simulink model "LR4_MostKran_1"  (R2019b)
settings: Solver=FixedStepAuto  StartTime=0.0  StopTime=70  FixedStep=dT  RelTol=1e-3  EnableMultiTasking=on
values from neighbouring files (symbols this model uses):
  A = [0, 1, 0, 0;  0, 0, a23, 0;  0, 0, 0, 1;  0, 0, a43, 0]    [LR_4_MostKran.m]
  B = [0; b2; 0; b4]    [LR_4_MostKran.m]
  C = [1, 0, 0, 0; 0, 1, 0, 0; 0, 0, 1, 0; 0, 0, 0, 1]    [LR_4_MostKran.m]
  D = [0; 0; 0; 0]    [LR_4_MostKran.m]
  fisREG = readfis('RgMostKran_1')    [LR_4_MostKran.m]
  KdE = 1/3    (= 0.333333333333)    [LR_4_MostKran.m]
  KEr = 1/40    (= 0.025)    [LR_4_MostKran.m]
  KU = 40    [LR_4_MostKran.m]
  X0 = [0; 0; 0; 0]    [LR_4_MostKran.m]
undefined symbols (not defined in the file or in its folder): sigbuilder_block
libraries: fuzblock x1
settings Model: Creator=Сергей  LastModifiedBy=danil
settings DataIOCC: LimitDataPoints=on  ReturnWorkspaceOutputs=off
settings OptimizationCC: LifeSpan=inf
settings DebuggingCC: AllowSymbolicDim=off  SFUnexpectedBacktrackingDiag=warning  SFNoUnconditionalDefaultTransitionDiag=warning  SFExecutionAtInitializationDiag=none  ArithmeticOperatorsInVariantConditions=warning
settings ModelReferenceCC: PropagateSignalLabelsOutOfModel=off
settings SFSimCC: SimUseLocalCustomCode=off  CustomCodeUndefinedFunction=UseInterfaceOnly
settings RTWCC: RTWUseLocalCustomCode=off
settings CodeAppCC: StateflowObjectComments=on
settings GRTTargetCC: TargetLangStandard=C89/C90 (ANSI)
settings ConfigComp: CovMetricSettings=dw  CovHtmlReporting=on  CovSaveCumulativeToWorkspaceVar=on  CovSaveSingleToWorkspaceVar=on  CovExternalEMLEnable=off

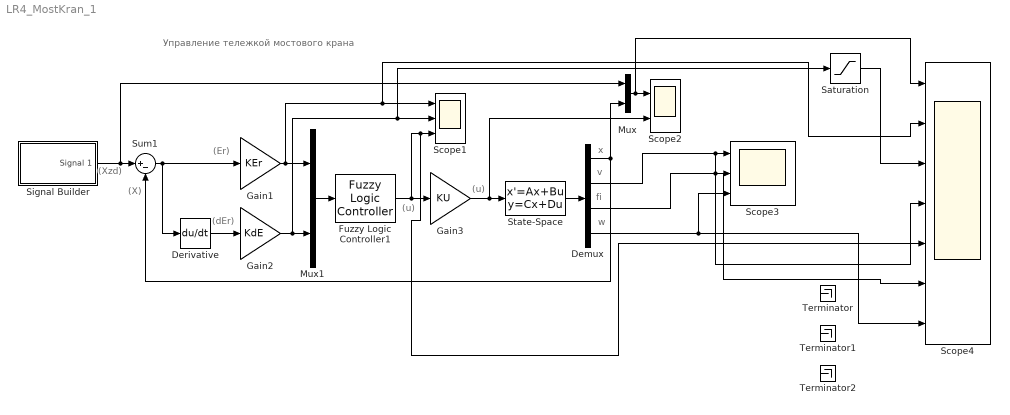
== system LR4_MostKran_1 ==
  note: w
  note: fi
  note: v
  note: x
  note: (Xzd)
  note: Управление тележкой мостового крана
  note: (Er)
  note: (dEr)
  note: (u)
  note: (u)
  note: (X)
  Demux : Demux
  Derivative : Derivative
  Fuzzy Logic Controller1 : fuzblock/Fuzzy Logic  Controller  FIS=[fisREG]  OutputSampleNumber=101  DataType=double  FuzzifiedInputs=off  RuleFiringStrengths=off  RuleOutputs=off  AggregatedOutputs=off  SimulateUsing=Interpreted execution  OutOfRangeInputValueMessage=warning  NoRuleFiredMessage=warning  EmptyOutputFuzzySetMessage=warning
  Gain1 : Gain  Gain=KEr
  Gain2 : Gain  Gain=KdE
  Gain3 : Gain  Gain=KU
  Mux : Mux  Inputs=2
  Mux1 : Mux  Inputs=2
  Saturation : Saturate  UpperLimit=1  LowerLimit=-1
  Scope1 : Scope  NumInputPorts=3
  Scope2 : Scope  NumInputPorts=2
  Scope3 : Scope  NumInputPorts=3
  Scope4 : Scope  NumInputPorts=7
  Signal Builder : Subsystem  Tag=STV Subsys  LoadFcn=sigbuilder_block('load');  StartFcn=sigbuilder_block('start');  StopFcn=sigbuilder_block('stop');  ClipboardFcn=sigbuilder_block('clipboard');  mask(Sigbuilder block){tuvar=[0:10]}
      mask help: Simulink:masks:SigbuilderBlock_MD
      mask init:
      | if ~strcmp(get_param(bdroot(gcbh),'SimulationStatus'),'stopped') tuvar = sigbuilder_block('maskInit'); end
      settings: CopyFcn=sigbuilder_block('copy');  DeleteFcn=sigbuilder_block('delete');  ModelCloseFcn=sigbuilder_block('modelClose');  PreSaveFcn=sigbuilder_block('preSave');  PauseFcn=sigbuilder_block('pause');  ContinueFcn=sigbuilder_block('continue');  NameChangeFcn=sigbuilder_block('namechange');  OpenFcn=sigbuilder_block('open',[63.75 114.75 550.5 399.75 ]);  CloseFcn=sigbuilder_block('close');
      mask Display: plot(0, 0, 100, 100,[2, 2, 32, 32, 2], [68, 8, 8, 68, 68],[32, 2], [38, 38], [32, 19, 2],[53, 60, 44], [32, 17, 17, 2],[16, 16, 31, 31]);txt = getActiveGroup(gcbh);text(2, 100, txt,'verticalAlignment', 'top');
  State-Space : StateSpace  A=A  B=B  C=C  D=D  InitialCondition=X0
  Sum1 : Sum  Inputs=|+-
  Terminator : Terminator
  Terminator1 : Terminator
  Terminator2 : Terminator
  wires:
  Signal Builder/1(Signal 1) -> Mux/1, Sum1/1
  State-Space/1 -> Demux/1
  Demux/1 -> Sum1/2, Mux/2
  Demux/2 -> Scope4/5, Scope3/1
  Demux/3 -> Scope4/6, Scope3/2
  Demux/4 -> Scope4/7, Scope3/3
  Mux1/1 -> Fuzzy Logic Controller1/1
  Sum1/1 -> Derivative/1, Gain1/1
  Gain1/1 -> Scope4/2, Scope1/1, Mux1/1
  Gain2/1 -> Saturation/1, Scope1/2, Mux1/2
  Mux/1 -> Scope4/1, Scope2/1
  Fuzzy Logic Controller1/1 -> Gain3/1, Scope4/4, Scope1/3
  Gain3/1 -> Scope2/2, State-Space/1
  Derivative/1 -> Gain2/1
  Saturation/1 -> Scope4/3

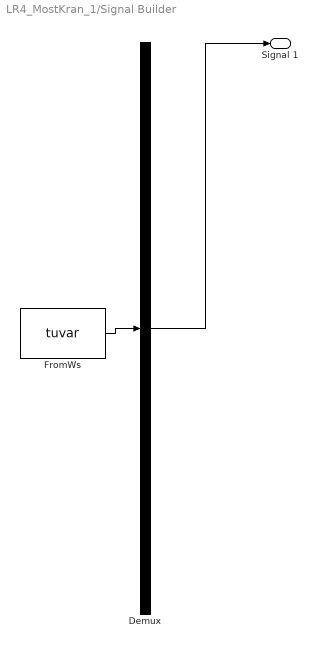
== system LR4_MostKran_1/Signal Builder ==
  Demux : Demux  Tag=STV Demux  Outputs=1
  FromWs : FromWorkspace  Tag=STV FromWs  VariableName=tuvar  SampleTime=0
      SigBuilderData=|
      | common.afterFinalStr = 'Extrapolate'
      | common.sampleTime = 0
      | dataSet.timeRange = [0 300]
      | dataSet.name = 'Group 1'
      | sbobj.Groups.Name = 'Group 1'
      | sbobj.Groups.Signals.Name = 'Signal 1'
      | sbobj.Groups.Signals.XData = [0 10 10 100 100 200 200 300]
      | sbobj.Groups.Signals.YData = [0 0 40 40 20 20 -0.2 -0.2]
      | sbobj.Groups.TimeRange = [0 300]
  Signal 1 : Outport  Tag=STV Outport
  wires:
  Demux/1 -> Signal 1/1
  FromWs/1 -> Demux/1
